simulink model "SplitFlightStats"  (R2020b)
settings: Solver=VariableStepAuto  StartTime=0.0  StopTime=10.0  RelTol=1e-3
libraries: aerolibv1 x1, visiontextngfix x1, visionsinks x1
settings Model: Creator=macra  LastModifiedBy=macra

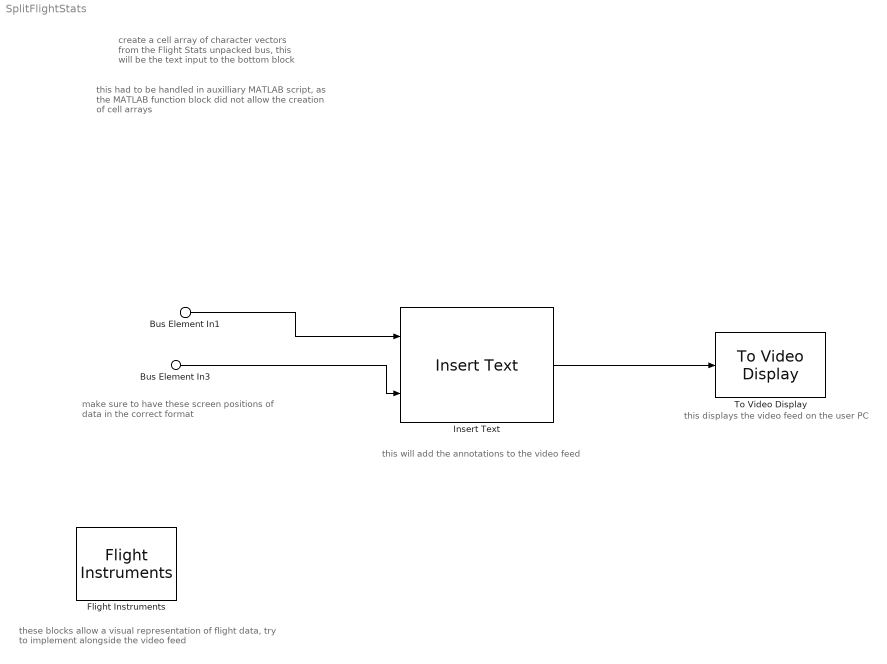
== system SplitFlightStats ==
  note: this had to be handled in auxilliary MATLAB script,
      | as the MATLAB function block did not allow the
      | creation of cell arrays
  note: these blocks allow a visual representation of flight data,
      | try to implement alongside the video feed
  note: this displays the video feed on the user PC
  note: this will add the annotations to the video feed
  note: make sure to have these screen positions of
      | data in the correct format
  note: create a cell array of character vectors
      | from the Flight Stats unpacked bus, this
      | will be the text input to the bottom block
  Bus Element In3 : Inport  PortName=Screen Postions of Data
  Bus Element In1 : Inport  Port=2  PortName=Camera Feed
  Flight Instruments : aerolibv1/Flight Instruments  SystemSampleTime=-1  VariantActivationTime=update diagram  Latency=0  AutoFrameSizeCalculation=off
      settings: SourceProductBaseCode=AE
  Insert Text : visiontextngfix/Insert Text  inputType=Obsolete  theText=FlightDataOutput  getTextLocFrom=Input port  textLoc=[1 1]  getTextColorFrom=Specify via dialog  textColor=[0 0 0]  getTextIntensityFrom=Specify via dialog  textIntensity=0  getTextOpacityFrom=Specify via dialog  textOpacity=1.0  dummyVar2=0  dummyVar3=0  dummyVar4=0  imagePorts=One multidimensional signal  isInputTransposed=off  fontFace=LucidaSansRegular  dummyVar1=0  blockFontSize=12  antiAliased=on
      settings: SourceProductBaseCode=VP
  To Video Display : visionsinks/To Video Display  windowSizeMode=Full-screen (Esc to exit)  openAtMdlStart=on  fullScreen=off  videoWindowX=536805376  videoWindowY=536805376  saveWindowSize=off  videoWindowWidth=2147483647  videoWindowHeight=2147483647  inputColorFormat=RGB  inputType=Obsolete  imagePorts=One multidimensional signal  OutputDevice=On-screen video monitor  dataOrg=Column-major  isWindowOpen=off
  wires:
  Bus Element In1/1 -> Insert Text/1
  Insert Text/1 -> To Video Display/1
  Bus Element In3/1 -> Insert Text/2
